simulink model "Clark"  (R2022b)
settings: Solver=ode4  StartTime=0.0  StopTime=10.0  FixedStep=1e-5  RelTol=1e-3
values from neighbouring files (symbols this model uses):
  Ts = 1/fs    (= 0.0001)    [FOCinit.m]
settings Model: Creator=ZinouAb  LastModifiedBy=ZinouAb

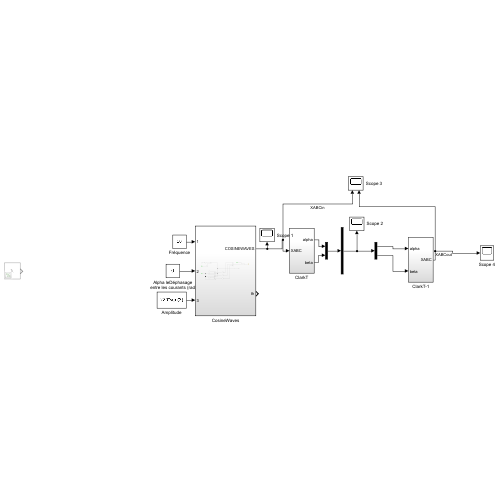
[thumbnail: Simulink's stored preview of the top-level diagram]
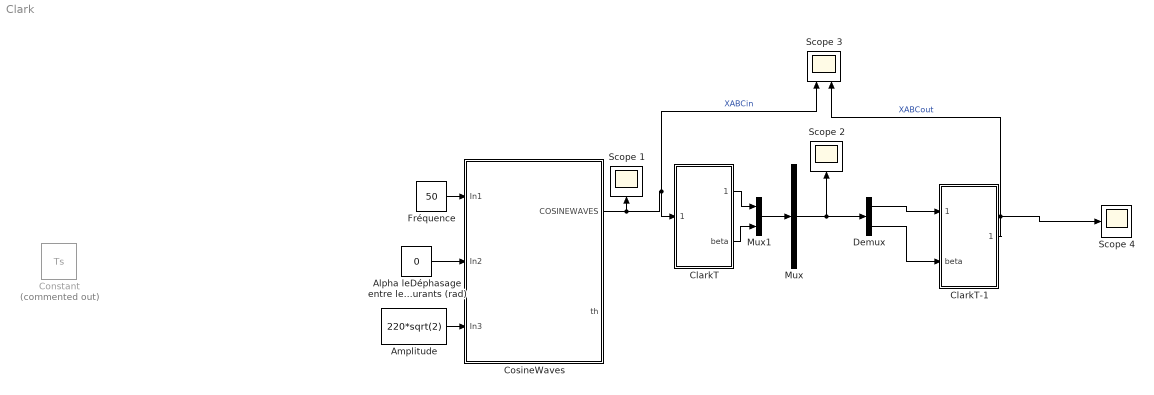
== system Clark ==
  Alpha leDéphasage entre les courants (rad) : Constant  Value=0
  Amplitude : Constant  Value=220*sqrt(2)
  ClarkT : Subsystem
  ClarkT-1 : Subsystem
  Constant : Constant  Commented=on  Value=Ts
  CosineWaves : Subsystem
  Demux : Demux  Outputs=2
  Fréquence : Constant  Value=50
  Mux : Mux  Inputs=1
  Mux1 : Mux  Inputs=2
  Scope 1 : Scope
  Scope 2 : Scope
  Scope 3 : Scope  NumInputPorts=2
  Scope 4 : Scope
  wires:
  Mux1/1 -> Mux/1
  Mux/1 -> Demux/1, Scope 2/1
  ClarkT-1/1(XABC) -> Scope 3/2, Scope 4/1  "XABCout"
  Amplitude/1 -> CosineWaves/3(In3)
  Alpha leDéphasage entre les courants (rad)/1 -> CosineWaves/2(In2)
  Fréquence/1 -> CosineWaves/1(In1)
  CosineWaves/1(COSINEWAVES) -> ClarkT/1(XABC), Scope 3/1, Scope 1/1  "XABCin"
  ClarkT/1(alpha) -> Mux1/1
  ClarkT/2(beta) -> Mux1/2
  Demux/1 -> ClarkT-1/1(alpha)
  Demux/2 -> ClarkT-1/2(beta)

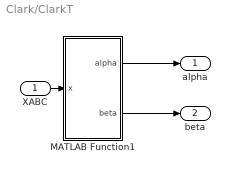
== system Clark/ClarkT ==
  XABC : Inport
  MATLAB Function1 : MATLAB Function  TreatAsAtomicUnit=on
  alpha : Outport
  beta : Outport  Port=2
  wires:
  MATLAB Function1/1(alpha) -> alpha/1
  XABC/1 -> MATLAB Function1/1(x)
  MATLAB Function1/2(beta) -> beta/1

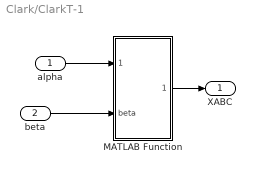
== system Clark/ClarkT-1 ==
  alpha : Inport
  beta : Inport  Port=2
  MATLAB Function : MATLAB Function  TreatAsAtomicUnit=on
  XABC : Outport
  wires:
  MATLAB Function/1(XABC) -> XABC/1
  alpha/1 -> MATLAB Function/1(alpha)
  beta/1 -> MATLAB Function/2(beta)

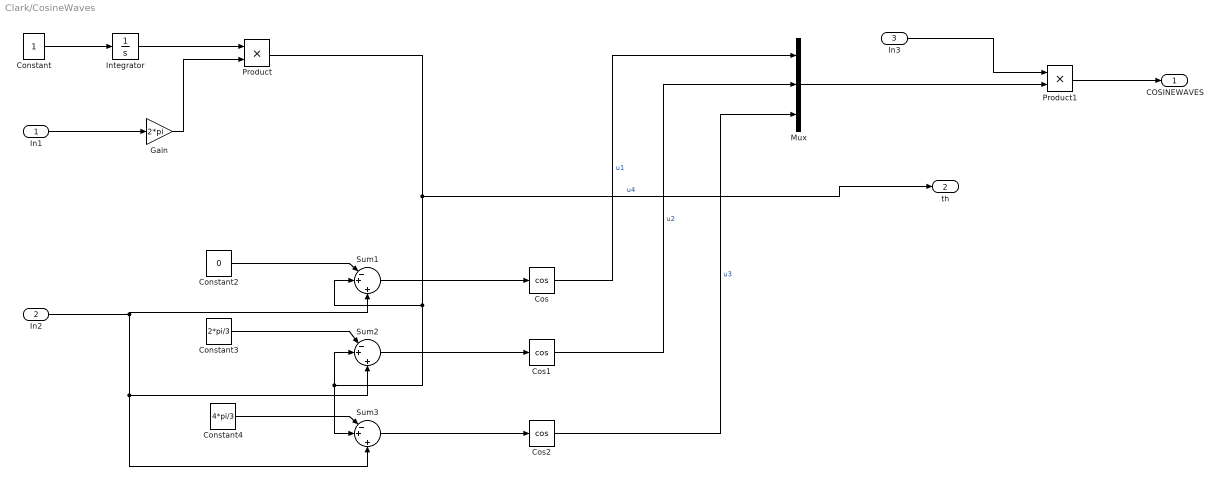
== system Clark/CosineWaves ==
  In1 : Inport
  In2 : Inport  Port=2
  In3 : Inport  Port=3
  Constant : Constant
  Constant2 : Constant  Value=0
  Constant3 : Constant  Value=2*pi/3
  Constant4 : Constant  Value=4*pi/3
  Cos : Trigonometry  Operator=cos
  Cos1 : Trigonometry  Operator=cos
  Cos2 : Trigonometry  Operator=cos
  Gain : Gain  Gain=2*pi
  Integrator : Integrator
  Mux : Mux  Inputs=3
  Product : Product
  Product1 : Product
  Sum1 : Sum  Inputs=|-+|+
  Sum2 : Sum  Inputs=|-+|+
  Sum3 : Sum  Inputs=|-+|+
  COSINEWAVES : Outport
  th : Outport  Port=2
  wires:
  Constant/1 -> Integrator/1
  Sum2/1 -> Cos1/1
  In2/1 -> Sum1/3, Sum3/3, Sum2/3
  Product/1 -> th/1, Sum3/2, Sum2/2, Sum1/2  "u4"
  Constant3/1 -> Sum2/1
  Sum3/1 -> Cos2/1
  Sum1/1 -> Cos/1
  Constant2/1 -> Sum1/1
  Constant4/1 -> Sum3/1
  Gain/1 -> Product/2
  Integrator/1 -> Product/1
  In1/1 -> Gain/1
  Cos1/1 -> Mux/2  "u2"
  Cos/1 -> Mux/1  "u1"
  Cos2/1 -> Mux/3  "u3"
  Mux/1 -> Product1/2
  In3/1 -> Product1/1
  Product1/1 -> COSINEWAVES/1

== matlab function Clark/ClarkT/MATLAB Function1 ==
  data: x input; alpha output; beta output
function [alpha,beta] = Clark(x)
P=(2/3)*[ cos(0) cos(0-2*pi/3) cos(0+2*pi/3);
         -sin(0) -sin(0-2*pi/3) -sin(0+2*pi/3)  ];
prod=P*x;
alpha=prod(1);
beta=prod(2);

== matlab function Clark/ClarkT-1/MATLAB Function ==
  data: alpha input; beta input; XABC output
function XABC= Clarkinv(alpha,beta)

parkinv = [ cos(0),           -sin(0); 
          cos(0-2*pi/3), -sin(0-2*pi/3); 
          cos(0+2*pi/3), -sin(0+2*pi/3)];

XABC = parkinv * [alpha;beta];

% x1=temp(1);
% x2=temp(2);
% x3=temp(3);
